simulink model "Async_3br_conv_eff"  (R2024b)
settings: Solver=ode23tb  StartTime=0.0  StopTime=10.5  MaxStep=1e-2  MinStep=1e-5  RelTol=1e-1
InitFcn:
  | sw_freq=60e3;
  | eff_rms_freq=sw_freq/10;
  | V_high=80;
  | 
  | L_ind=300e-6;
  | L_res=20e-3;
  | 
  | MOS_Ron=10e-3;
  | MOS_Vfw=1.2;
  | 
  | DIO_Vfw=0.9;
  | DIO_Ron=1e-3;
  | 
  | TRC_Res=5e-3;
  | 
  | sync_mode=1;
  | 
  | asym_bdc_p=0.01;
  | asym_bdc_i=0.8;
values from neighbouring files (symbols this model uses):
  runtime = 1.5    [compare_3d_br_ratios.m]
  timestep = runtime/size(curr_range,2)    [compare_3d_br_ratios.m]
  V_low_range = 10:5:40    [compare_3d_br_ratios.m]
undefined symbols (not defined in the file or in its folder): ratio
libraries: spsMeanLib x7, spsGroundLib x7, spsSeriesRLCBranchLib x7, slpidlib x4, spsMosfetLib x4, spsDiodeLib x2, spsStairGeneratorLib x2, spsMultimeterLib x1, spsDCVoltageSourceLib x1, spsControlledVoltageSourceLib x1, embmathops x1, spspowerguiLib x1
settings Model: SimulationMode=rapid-accelerator  Creator=adamo  LastModifiedBy=adamo
settings DebuggingCC: MaskedZcDiagnostic=none  IgnoredZcDiagnostic=none
settings HardwareCC: ProdHWDeviceType=AMD->x86-64 (Windows64)
settings RTWCC: BuildConfiguration=Faster Runs  CheckMdlBeforeBuild=Error
settings GRTTargetCC: OptimizeReductions=on
settings SimscapeCC: SimscapeCompileComponentReuse=on  SimscapeCompileArtifactsDiskCache=on

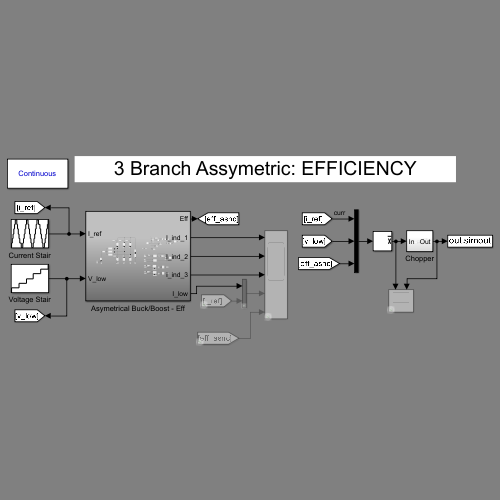
[thumbnail: Simulink's stored preview of the top-level diagram]
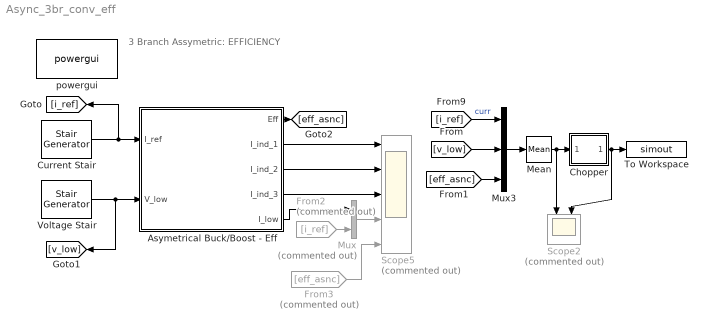
== system Async_3br_conv_eff ==
  note: 3 Branch Assymetric: EFFICIENCY
  Asymetrical Buck/Boost - Eff : Subsystem
  Chopper : Subsystem
  Current Stair : spsStairGeneratorLib/Stair Generator  t=cur_stair_time  e=current_stair  Ts=0
  From2 : From  Commented=on  GotoTag=i_ref
  From3 : From  Commented=on  GotoTag=eff_asnc
  Mean : spsMeanLib/Mean  Freq=sw_freq/10  Vinit=0  Ts=0
  Mux : Mux  Commented=on  Inputs=2
  Mux3 : Mux  Inputs=3
  Scope2 : Scope  Commented=on  NumInputPorts=2
  Scope5 : Scope  Commented=on  NumInputPorts=5
  To Workspace : ToWorkspace  VariableName=simout  SampleTime=-1
  Voltage Stair : spsStairGeneratorLib/Stair Generator  t=[0:runtime:runtime*length(V_low_range)-runtime]  e=V_low_range  Ts=0
  powergui : spspowerguiLib/powergui  Priority=1  SimulationMode=Continuous  SampleTime=50e-6  frequency=60  Iterations=50  frequencyindice=0  Pbase=100e6  ErrMax=1e-4  UnitsV=kV  UnitsW=MW  buscounter=0  FunctionMessages=off  echomessages=off  EnableUseOfTLC=off  CurrentSourceSwitches=off  DisableSnubberDevices=on  DisableRonSwitches=off  DisableVfSwitches=off  DisplayEquations=off  AutomaticDiscreteSolvers=off  SolverType=Tustin/Backward Euler (TBE)  Interpol=off  ExternalGateDelay=off  methode=on  Ts=100  x0status=blocks  SPID=on  SwTol=0  HookPort=off  NonlinearTolerance=1e-4  nMaxIteration=100  ContinueOnMaxIteration=off  RestoreLinks=warning  ResistiveCurrentMeasurement=off  Frange=[0:2:500]  Ylog=off  Xlog=on  ShowGrid=off  save=off  variable=ZData  structure=0  ZoomFFT=off  StartTime=0.0  cycles=1  DisplayStyle=1  fundamental=60  FreqAxis=off  MaxFrequency=1000  frequencyindicesteady=1  RmsSteady=1  display=off
  wires:
  Current Stair/1 -> [i_ref], Asymetrical Buck/Boost - Eff/1(I_ref)
  Asymetrical Buck/Boost - Eff/2(I_ind_1) -> Scope5/1
  Asymetrical Buck/Boost - Eff/3(I_ind_2) -> Scope5/2
  Asymetrical Buck/Boost - Eff/4(I_ind_3) -> Scope5/3
  Asymetrical Buck/Boost - Eff/1(Eff) -> [eff_asnc]
  [i_ref] -> Mux3/1  "curr"
  Mux3/1 -> Mean/1
  [eff_asnc] -> Mux3/3
  Asymetrical Buck/Boost - Eff/5(I_low) -> Mux/1
  Chopper/1(Out1) -> Scope2/2, To Workspace/1
  Mean/1 -> Scope2/1, Chopper/1(In1)
  Voltage Stair/1 -> [v_low], Asymetrical Buck/Boost - Eff/2(V_low)
  [v_low] -> Mux3/2
  Mux/1 -> Scope5/4
  From2/1 -> Mux/2
  From3/1 -> Scope5/5

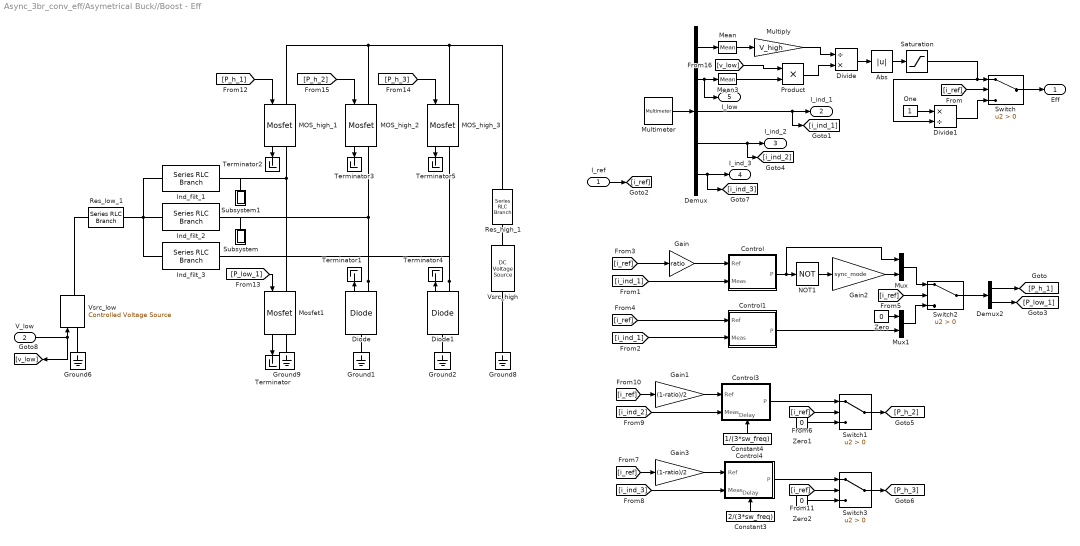
== system Async_3br_conv_eff/Asymetrical Buck//Boost - Eff ==
  I_ref : Inport
  V_low : Inport  Port=2
  Abs : Abs  SaturateOnIntegerOverflow=off
  Constant3 : Constant  Value=2/(3*sw_freq)
  Constant4 : Constant  Value=1/(3*sw_freq)
  Control : Subsystem
  Control1 : Subsystem
  Control3 : Subsystem
      settings: PortSchema="{\"entries\":[{\"content\":{\"sides\":[{\"content\":{\"connectorIds\":[\"In1\",\"In2\"]},\"type\":\"ConnectorPlacement.EquallySpacedRectSide\",\"uuid\":\"44975c06-6cb3-4b92-aa2e-c11b859d13e4\"},{\"content\":{\"connectorIds\":[\"Out1\"],\"side\":\"RIGHT\"},\"type\":\"ConnectorPlacement.EquallySpacedRectSide\",\"uuid\":\"ebdc9065-5b19-4aa7-8841-916fd82a5d31\"},{\"content\":{\"side\":\"TOP\"},\"type\":\"ConnectorPlacement.EquallySpacedRectSide\",\"uuid\":\"027925ea-888b-4bcf-b8a4-44694d0e275e\"},{\"content\":{\"connectorIds\":[\"In3\"],\"side\":\"BOTTOM\"},\"type\":\"ConnectorPlacement.EquallySpacedRectSide\",\"uuid\":\"415fb0af-dd9a-4309-9118-76332ed11379\"}]},\"type\":\"ConnectorPlacement.EquallySpacedConnector\",\"uuid\":\"3cd19595-535e-42c3-a0e6-40045bedee28\"}],\"packageUris\":[\"http://schema.mathworks.com/mf0/Connector/R2020b\"],\"version\":\"1.0\"}"
  Control4 : Subsystem
      settings: PortSchema="{\"entries\":[{\"content\":{\"sides\":[{\"content\":{\"connectorIds\":[\"In1\",\"In2\"]},\"type\":\"ConnectorPlacement.EquallySpacedRectSide\",\"uuid\":\"44975c06-6cb3-4b92-aa2e-c11b859d13e4\"},{\"content\":{\"connectorIds\":[\"Out1\"],\"side\":\"RIGHT\"},\"type\":\"ConnectorPlacement.EquallySpacedRectSide\",\"uuid\":\"ebdc9065-5b19-4aa7-8841-916fd82a5d31\"},{\"content\":{\"side\":\"TOP\"},\"type\":\"ConnectorPlacement.EquallySpacedRectSide\",\"uuid\":\"027925ea-888b-4bcf-b8a4-44694d0e275e\"},{\"content\":{\"connectorIds\":[\"In3\"],\"side\":\"BOTTOM\"},\"type\":\"ConnectorPlacement.EquallySpacedRectSide\",\"uuid\":\"9488b47a-c58c-42e9-bacd-7bb9f563b775\"}]},\"type\":\"ConnectorPlacement.EquallySpacedConnector\",\"uuid\":\"3cd19595-535e-42c3-a0e6-40045bedee28\"}],\"packageUris\":[\"http://schema.mathworks.com/mf0/Connector/R2020b\"],\"version\":\"1.0\"}"
  Demux : Demux  Outputs=5
  Demux2 : Demux  Outputs=2
  Diode : spsDiodeLib/Diode  Ron=DIO_Ron  Lon=0  Vf=DIO_Vfw  IC=0  UseSnubber=0  Rs=500  Cs=250e-9  Measurements=on
  Diode1 : spsDiodeLib/Diode  Ron=DIO_Ron  Lon=0  Vf=DIO_Vfw  IC=0  UseSnubber=0  Rs=500  Cs=250e-9  Measurements=on
  Divide : Product  Inputs=/*
  Divide1 : Product  Inputs=*/
  Gain : Gain  Gain=ratio
  Gain1 : Gain  Gain=(1-ratio)/2
  Gain2 : Gain  Gain=sync_mode  OutDataTypeStr=double
  Gain3 : Gain  Gain=(1-ratio)/2
  Ground{1..2,6,8..9} (5 alike) : spsGroundLib/Ground  LConnTagsString=a
  Ind_filt_1 : spsSeriesRLCBranchLib/Series RLC Branch  LConnTagsString=__new0  RConnTagsString=__new0  BranchType=RL  Resistance=L_res  Inductance=L_ind  SetiL0=off  InitialCurrent=0  Capacitance=1e-6  Setx0=off  InitialVoltage=0  Measurements=Branch current
  Ind_filt_2 : spsSeriesRLCBranchLib/Series RLC Branch  LConnTagsString=__new0  RConnTagsString=__new0  BranchType=RL  Resistance=L_res  Inductance=L_ind  SetiL0=off  InitialCurrent=0  Capacitance=1e-6  Setx0=off  InitialVoltage=0  Measurements=Branch current
  Ind_filt_3 : spsSeriesRLCBranchLib/Series RLC Branch  LConnTagsString=__new0  RConnTagsString=__new0  BranchType=RL  Resistance=L_res  Inductance=L_ind  SetiL0=off  InitialCurrent=0  Capacitance=1e-6  Setx0=off  InitialVoltage=0  Measurements=Branch current
  MOS_high_1 : spsMosfetLib/Mosfet  Ron=MOS_Ron  Lon=0  Rd=DIO_Ron  Vfd=MOS_Vfw  IC=0  Rs=1e5  Cs=inf  Measurements=on
  MOS_high_2 : spsMosfetLib/Mosfet  Ron=MOS_Ron  Lon=0  Rd=DIO_Ron  Vfd=MOS_Vfw  IC=0  Rs=1e5  Cs=inf  Measurements=on
  MOS_high_3 : spsMosfetLib/Mosfet  Ron=MOS_Ron  Lon=0  Rd=DIO_Ron  Vfd=MOS_Vfw  IC=0  Rs=1e5  Cs=inf  Measurements=on
  Mean : spsMeanLib/Mean  Freq=eff_rms_freq  Vinit=1  Ts=0
  Mean3 : spsMeanLib/Mean  Freq=eff_rms_freq  Vinit=1  Ts=0
  Mosfet1 : spsMosfetLib/Mosfet  Ron=MOS_Ron  Lon=0  Rd=DIO_Ron  Vfd=MOS_Vfw  IC=0  Rs=1e5  Cs=inf  Measurements=on
  Multimeter : spsMultimeterLib/Multimeter  L=5  sel=[4 5 1 2 3]  yselected={}  Gain=[1 1 1 1 1]  OutputType=Complex  PlotAtSimulationStop=off  PhasorSimulation=off
  Multiply : Gain  Gain=V_high
  Mux : Mux  Inputs=2
  Mux1 : Mux  Inputs=2
  NOT1 : Logic  Operator=NOT  IconShape=distinctive  AllPortsSameDT=off  OutDataTypeStr=boolean
  One : Constant  OutDataTypeStr=Inherit: Inherit via back propagation
  Product : Product
  Res_high_1 : spsSeriesRLCBranchLib/Series RLC Branch  LConnTagsString=__new0  RConnTagsString=__new0  BranchType=R  Resistance=TRC_Res  Inductance=1e-3  SetiL0=off  InitialCurrent=0  Capacitance=1e-6  Setx0=off  InitialVoltage=0  Measurements=Branch current
  Res_low_1 : spsSeriesRLCBranchLib/Series RLC Branch  LConnTagsString=__new0  RConnTagsString=__new0  BranchType=R  Resistance=TRC_Res  Inductance=1e-3  SetiL0=off  InitialCurrent=0  Capacitance=1e-6  Setx0=off  InitialVoltage=0  Measurements=Branch current
  Saturation : Saturate  UpperLimit=0.9999  LowerLimit=0.4
  Subsystem : Subsystem
      settings: PortSchema="{\"entries\":[{\"content\":{\"sides\":[{\"content\":{},\"type\":\"ConnectorPlacement.EquallySpacedRectSide\",\"uuid\":\"333a472d-5660-403e-9749-9e5a485a4e51\"},{\"content\":{\"side\":\"RIGHT\"},\"type\":\"ConnectorPlacement.EquallySpacedRectSide\",\"uuid\":\"46e3a3df-9b43-4056-bf49-6d97e0ff375e\"},{\"content\":{\"connectorIds\":[\"LConn1\"],\"side\":\"TOP\"},\"type\":\"ConnectorPlacement.EquallySpacedRectSide\",\"uuid\":\"a9be43b9-3284-437d-b483-2a714199e3a2\"}]},\"type\":\"ConnectorPlacement.EquallySpacedConnector\",\"uuid\":\"6030dd83-63ea-4a67-9f73-95d000b3af89\"}],\"packageUris\":[\"http://schema.mathworks.com/mf0/Connector/R2020b\"],\"version\":\"1.0\"}"
  Subsystem1 : Subsystem
      settings: PortSchema="{\"entries\":[{\"content\":{\"sides\":[{\"content\":{},\"type\":\"ConnectorPlacement.EquallySpacedRectSide\",\"uuid\":\"333a472d-5660-403e-9749-9e5a485a4e51\"},{\"content\":{\"side\":\"RIGHT\"},\"type\":\"ConnectorPlacement.EquallySpacedRectSide\",\"uuid\":\"46e3a3df-9b43-4056-bf49-6d97e0ff375e\"},{\"content\":{\"connectorIds\":[\"LConn1\"],\"side\":\"TOP\"},\"type\":\"ConnectorPlacement.EquallySpacedRectSide\",\"uuid\":\"a9be43b9-3284-437d-b483-2a714199e3a2\"}]},\"type\":\"ConnectorPlacement.EquallySpacedConnector\",\"uuid\":\"6030dd83-63ea-4a67-9f73-95d000b3af89\"}],\"packageUris\":[\"http://schema.mathworks.com/mf0/Connector/R2020b\"],\"version\":\"1.0\"}"
  Switch{,1..3} (4 alike) : Switch  Criteria=u2 > Threshold  SaturateOnIntegerOverflow=off  InputSameDT=off
  Terminator{,1..5} (6 alike) : Terminator
  Vsrc_high : spsDCVoltageSourceLib/DC Voltage Source  Amplitude=V_high  Measurements=None
  Vsrc_low : spsControlledVoltageSourceLib/Controlled Voltage Source  Initialize=on  Source_Type=DC  Amplitude=10  Phase=0  Frequency=0  Measurements=None
  Zero : Constant  Value=0  OutDataTypeStr=Inherit: Inherit via back propagation
  Zero1 : Constant  Value=0  OutDataTypeStr=Inherit: Inherit via back propagation
  Zero2 : Constant  Value=0  OutDataTypeStr=Inherit: Inherit via back propagation
  Eff : Outport
  I_ind_1 : Outport  Port=2
  I_ind_2 : Outport  Port=3
  I_ind_3 : Outport  Port=4
  I_low : Outport  Port=5
  wires:
  [P_h_1] -> MOS_high_1/1
  MOS_high_1/1 -> Terminator2/1
  Mosfet1/1 -> Terminator/1
  [P_low_1] -> Mosfet1/1
  Diode/1 -> Terminator1/1
  MOS_high_2/1 -> Terminator3/1
  Diode1/1 -> Terminator4/1
  MOS_high_3/1 -> Terminator5/1
  [P_h_3] -> MOS_high_3/1
  Multimeter/1 -> Demux/1
  One/1 -> Divide1/1
  Mean/1 -> Multiply/1
  Divide1/1 -> Switch/3
  Saturation/1 -> Divide1/2, Switch/1
  Divide/1 -> Abs/1
  Switch/1 -> Eff/1
  Abs/1 -> Saturation/1
  Control/1(P) -> Mux/1, NOT1/1
  [i_ref] -> Gain/1
  Switch2/1 -> Demux2/1
  Mux/1 -> Switch2/1
  [i_ind_1] -> Control/2(Meas)
  Demux2/2 -> [P_low_1]
  Demux2/1 -> [P_h_1]
  Gain2/1 -> Mux/2
  [i_ref] -> Switch2/2
  I_ref/1 -> [i_ref]
  [i_ref] -> Switch/2
  NOT1/1 -> Gain2/1
  [P_h_2] -> MOS_high_2/1
  Gain/1 -> Control/1(Ref)
  [i_ref] -> Control1/1(Ref)
  [i_ind_1] -> Control1/2(Meas)
  Control1/1(P) -> Mux1/2
  Mean3/1 -> Product/2
  Demux/1 -> Mean/1
  Demux/2 -> I_low/1, Mean3/1
  Demux/5 -> [i_ind_3], I_ind_3/1
  Demux/4 -> [i_ind_2], I_ind_2/1
  Demux/3 -> [i_ind_1], I_ind_1/1
  Product/1 -> Divide/2
  Multiply/1 -> Divide/1
  Mux1/1 -> Switch2/3
  Zero/1 -> Mux1/1
  Constant4/1 -> Control3/3(Delay)
  Constant3/1 -> Control4/3(Delay)
  [i_ref] -> Gain1/1
  Gain1/1 -> Control3/1(Ref)
  [i_ind_2] -> Control3/2(Meas)
  Control3/1(P) -> Switch1/1
  Switch1/1 -> [P_h_2]
  Zero1/1 -> Switch1/3
  [i_ref] -> Switch1/2
  [i_ind_3] -> Control4/2(Meas)
  [i_ref] -> Switch3/2
  Control4/1(P) -> Switch3/1
  Switch3/1 -> [P_h_3]
  Zero2/1 -> Switch3/3
  V_low/1 -> [v_low], Vsrc_low/1
  [v_low] -> Product/1
  [i_ref] -> Gain3/1
  Gain3/1 -> Control4/1(Ref)
  connections:
  Diode/RConn1 -- Ind_filt_2/LConn1 -- Subsystem/LConn1 -- MOS_high_2/RConn1
  MOS_high_1/RConn1 -- Subsystem1/LConn1 -- Ind_filt_1/LConn1 -- Mosfet1/LConn1
  Ground8/LConn1 -- Vsrc_high/LConn1
  Mosfet1/RConn1 -- Ground9/LConn1
  Vsrc_low/LConn1 -- Ground6/LConn1
  Diode/LConn1 -- Ground1/LConn1
  Diode1/RConn1 -- Ind_filt_3/LConn1 -- MOS_high_3/RConn1
  Diode1/LConn1 -- Ground2/LConn1
  Vsrc_low/RConn1 -- Res_low_1/RConn1
  Res_high_1/LConn1 -- Vsrc_high/RConn1
  Ind_filt_2/RConn1 -- Res_low_1/LConn1 -- Ind_filt_3/RConn1 -- Ind_filt_1/RConn1
  Res_high_1/RConn1 -- MOS_high_1/LConn1 -- MOS_high_2/LConn1 -- MOS_high_3/LConn1

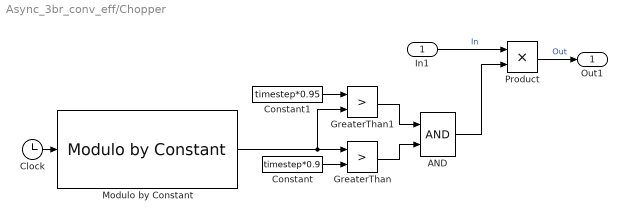
== system Async_3br_conv_eff/Chopper ==
  In1 : Inport
  AND : Logic  IconShape=distinctive  AllPortsSameDT=off  OutDataTypeStr=boolean
  Clock : Clock
  Constant : Constant  Value=timestep*0.9
  Constant1 : Constant  Value=timestep*0.95
  GreaterThan : RelationalOperator  Operator=>  OutDataTypeStr=boolean  RndMeth=Simplest  InputSameDT=off
  GreaterThan1 : RelationalOperator  Operator=>  OutDataTypeStr=boolean  RndMeth=Simplest  InputSameDT=off
  Modulo by Constant : embmathops/Modulo by Constant  Denominator=timestep  SimulateUsing=Code generation
  Product : Product
  Out1 : Outport
  wires:
  Clock/1 -> Modulo by Constant/1
  Constant/1 -> GreaterThan/2
  GreaterThan1/1 -> AND/1
  GreaterThan/1 -> AND/2
  AND/1 -> Product/2
  Modulo by Constant/1 -> GreaterThan1/2, GreaterThan/1
  Constant1/1 -> GreaterThan1/1
  In1/1 -> Product/1  "In"
  Product/1 -> Out1/1  "Out"

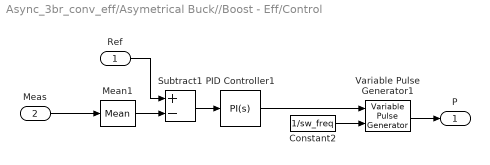
== system Async_3br_conv_eff/Asymetrical Buck//Boost - Eff/Control ==
  Ref : Inport
  Meas : Inport  Port=2
  Constant2 : Constant  Value=1/sw_freq
  Mean1 : spsMeanLib/Mean  Freq=sw_freq/10  Vinit=0  Ts=0
  PID Controller1 : slpidlib/PID Controller  Controller=PI  Form=Parallel  TimeDomain=Continuous-time  UseExternalTs=off  SampleTime=-1  IntegratorMethod=Forward Euler  FilterMethod=Forward Euler  ControllerParametersSource=internal  P=asym_bdc_p  I=asym_bdc_i  UseKiTs=on  D=0  UseExternalDerivativeSource=off  N=100  UseFilter=on  TunerSelectOption=Transfer Function Based (PID Tuner App)  InitialConditionSource=internal  InitialConditionForIntegrator=0.15  InitialConditionForFilter=0.1  DifferentiatorICPrevScaledInput=0  ExternalReset=none  TrackingMode=off  Kt=1  LimitOutput=on  SatLimitsSource=internal  UpperSaturationLimit=1  LowerSaturationLimit=0.01  LinearizeAsGain=on  AntiWindupMode=none  Kb=1  LimitIntegrator=off  UpperIntegratorSaturationLimit=inf  LowerIntegratorSaturationLimit=-inf  POutMin=[]  POutMax=[]  IOutMin=[]  IOutMax=[]  DOutMin=[]  DOutMax=[]  NOutMin=[]  NOutMax=[]  SumOutMin=[]  SumOutMax=[]  SaturationOutMin=[]  SaturationOutMax=[]  PParamMin=[]  PParamMax=[]  IParamMin=[]  IParamMax=[]  DParamMin=[]  DParamMax=[]  NParamMin=[]  NParamMax=[]  KbParamMin=[]  KbParamMax=[]  KtParamMin=[]  KtParamMax=[]  KbOutMin=[]  KbOutMax=[]  KtOutMin=[]  KtOutMax=[]  IntegratorOutMin=[]  IntegratorOutMax=[]  FilterOutMin=[]  FilterOutMax=[]  SumI1OutMin=[]  SumI1OutMax=[]  SumI2OutMin=[]  SumI2OutMax=[]  SumI3OutMin=[]  SumI3OutMax=[]  SumI4OutMin=[]  SumI4OutMax=[]  SumDOutMin=[]  SumDOutMax=[]  DifferentiatorOutMin=[]  DifferentiatorOutMax=[]  FilterDiffOutCoefMin=[]  FilterDiffOutCoefMax=[]  ReciprocalOutMin=[]  ReciprocalOutMax=[]  SumDenOutMin=[]  SumDenOutMax=[]  SumNumOutMin=[]  SumNumOutMax=[]  DivideOutMin=[]  DivideOutMax=[]  UdiffTsProdOutMin=[]  UdiffTsProdOutMax=[]  NTsProdOutMin=[]  NTsProdOutMax=[]  UintegralTsProdOutMin=[]  UintegralTsProdOutMax=[]  UngainTsProdOutMin=[]  UngainTsProdOutMax=[]  ClampingZeroOutDataTypeStr=Inherit: Inherit via back propagation  ClampingZeroOutMin=[]  ClampingZeroOutMax=[]  FilterDenConstantOutDataTypeStr=Inherit: Inherit via back propagation  FilterDenConstantOutMin=[]  FilterDenConstantOutMax=[]  PCopyOutDataTypeStr=Inherit: Inherit via back propagation  PCopyOutMin=[]  PCopyOutMax=[]  NCopyOutDataTypeStr=Inherit: Inherit via back propagation  NCopyOutMin=[]  NCopyOutMax=[]  IntegratorContinuousStateAttributes=''  IntegratorStateMustResolveToSignalObject=off  IntegratorRTWStateStorageClass=Auto  FilterContinuousStateAttributes=''  FilterStateMustResolveToSignalObject=off  FilterRTWStateStorageClass=Auto  ParallelPVariant=InternalParameters  IdealPVariant=Disabled  IVariant=InternalParameters  DVariant=Disabled  IntegratorVariant=Continuous  SatVariant=Enabled  AWVariant=Passthrough  PCopyVariant=Disabled  TRVariant=Disabled  FdbkBlocksVariant=Forward  IdealPFdbkVariant=Disabled  SatFdbkVariant=Disabled  DerivativeFilterVariant=Disabled  NVariant=Disabled  NCopyVariant=Disabled_SignalSpec  FilterICVariant=Disabled  IntegratorICVariant=InternalICs  ExternalResetVariant=Disabled  TRSumVariant=Passthrough  SumFdbkVariant=Disabled  SumVariant=Sum_PI  TsampFilterVariant=InternalTs  TsampNgainVariant=Passthrough  TsampIntegralVariant=Disabled_SignalSpec  ExternalSaturationOutDataTypeStr=Inherit: Same as second input  DerivativeSourceVariant=Disabled  PreIntVariant=InternalPreInt
  Subtract1 : Sum  Inputs=+-
  Variable Pulse Generator1 : VariablePulseGenerator  AllowZeroPulseWidth=on  SampleTime=0.1
  P : Outport
  wires:
  Meas/1 -> Mean1/1
  PID Controller1/1 -> Variable Pulse Generator1/1
  Constant2/1 -> Variable Pulse Generator1/2
  Mean1/1 -> Subtract1/2
  Subtract1/1 -> PID Controller1/1
  Variable Pulse Generator1/1 -> P/1
  Ref/1 -> Subtract1/1

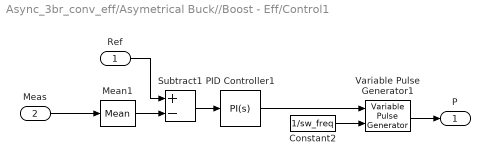
== system Async_3br_conv_eff/Asymetrical Buck//Boost - Eff/Control1 ==
  Ref : Inport
  Meas : Inport  Port=2
  Constant2 : Constant  Value=1/sw_freq
  Mean1 : spsMeanLib/Mean  Freq=sw_freq/10  Vinit=0  Ts=0
  PID Controller1 : slpidlib/PID Controller  Controller=PI  Form=Parallel  TimeDomain=Continuous-time  UseExternalTs=off  SampleTime=-1  IntegratorMethod=Forward Euler  FilterMethod=Forward Euler  ControllerParametersSource=internal  P=asym_bdc_p  I=asym_bdc_i  UseKiTs=on  D=0  UseExternalDerivativeSource=off  N=100  UseFilter=on  TunerSelectOption=Transfer Function Based (PID Tuner App)  InitialConditionSource=internal  InitialConditionForIntegrator=0  InitialConditionForFilter=0  DifferentiatorICPrevScaledInput=0  ExternalReset=none  TrackingMode=off  Kt=1  LimitOutput=on  SatLimitsSource=internal  UpperSaturationLimit=1  LowerSaturationLimit=0  LinearizeAsGain=on  AntiWindupMode=none  Kb=1  LimitIntegrator=off  UpperIntegratorSaturationLimit=inf  LowerIntegratorSaturationLimit=-inf  POutMin=[]  POutMax=[]  IOutMin=[]  IOutMax=[]  DOutMin=[]  DOutMax=[]  NOutMin=[]  NOutMax=[]  SumOutMin=[]  SumOutMax=[]  SaturationOutMin=[]  SaturationOutMax=[]  PParamMin=[]  PParamMax=[]  IParamMin=[]  IParamMax=[]  DParamMin=[]  DParamMax=[]  NParamMin=[]  NParamMax=[]  KbParamMin=[]  KbParamMax=[]  KtParamMin=[]  KtParamMax=[]  KbOutMin=[]  KbOutMax=[]  KtOutMin=[]  KtOutMax=[]  IntegratorOutMin=[]  IntegratorOutMax=[]  FilterOutMin=[]  FilterOutMax=[]  SumI1OutMin=[]  SumI1OutMax=[]  SumI2OutMin=[]  SumI2OutMax=[]  SumI3OutMin=[]  SumI3OutMax=[]  SumI4OutMin=[]  SumI4OutMax=[]  SumDOutMin=[]  SumDOutMax=[]  DifferentiatorOutMin=[]  DifferentiatorOutMax=[]  FilterDiffOutCoefMin=[]  FilterDiffOutCoefMax=[]  ReciprocalOutMin=[]  ReciprocalOutMax=[]  SumDenOutMin=[]  SumDenOutMax=[]  SumNumOutMin=[]  SumNumOutMax=[]  DivideOutMin=[]  DivideOutMax=[]  UdiffTsProdOutMin=[]  UdiffTsProdOutMax=[]  NTsProdOutMin=[]  NTsProdOutMax=[]  UintegralTsProdOutMin=[]  UintegralTsProdOutMax=[]  UngainTsProdOutMin=[]  UngainTsProdOutMax=[]  ClampingZeroOutDataTypeStr=Inherit: Inherit via back propagation  ClampingZeroOutMin=[]  ClampingZeroOutMax=[]  FilterDenConstantOutDataTypeStr=Inherit: Inherit via back propagation  FilterDenConstantOutMin=[]  FilterDenConstantOutMax=[]  PCopyOutDataTypeStr=Inherit: Inherit via back propagation  PCopyOutMin=[]  PCopyOutMax=[]  NCopyOutDataTypeStr=Inherit: Inherit via back propagation  NCopyOutMin=[]  NCopyOutMax=[]  IntegratorContinuousStateAttributes=''  IntegratorStateMustResolveToSignalObject=off  IntegratorRTWStateStorageClass=Auto  FilterContinuousStateAttributes=''  FilterStateMustResolveToSignalObject=off  FilterRTWStateStorageClass=Auto  ParallelPVariant=InternalParameters  IdealPVariant=Disabled  IVariant=InternalParameters  DVariant=Disabled  IntegratorVariant=Continuous  SatVariant=Enabled  AWVariant=Passthrough  PCopyVariant=Disabled  TRVariant=Disabled  FdbkBlocksVariant=Forward  IdealPFdbkVariant=Disabled  SatFdbkVariant=Disabled  DerivativeFilterVariant=Disabled  NVariant=Disabled  NCopyVariant=Disabled_SignalSpec  FilterICVariant=Disabled  IntegratorICVariant=InternalICs  ExternalResetVariant=Disabled  TRSumVariant=Passthrough  SumFdbkVariant=Disabled  SumVariant=Sum_PI  TsampFilterVariant=InternalTs  TsampNgainVariant=Passthrough  TsampIntegralVariant=Disabled_SignalSpec  ExternalSaturationOutDataTypeStr=Inherit: Same as second input  DerivativeSourceVariant=Disabled  PreIntVariant=InternalPreInt
  Subtract1 : Sum  Inputs=+-
  Variable Pulse Generator1 : VariablePulseGenerator  AllowZeroPulseWidth=on  SampleTime=0.1
  P : Outport
  wires:
  Meas/1 -> Mean1/1
  PID Controller1/1 -> Variable Pulse Generator1/1
  Constant2/1 -> Variable Pulse Generator1/2
  Mean1/1 -> Subtract1/2
  Subtract1/1 -> PID Controller1/1
  Variable Pulse Generator1/1 -> P/1
  Ref/1 -> Subtract1/1

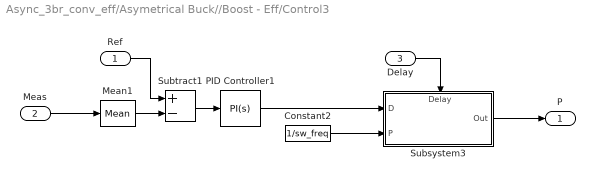
== system Async_3br_conv_eff/Asymetrical Buck//Boost - Eff/Control3 ==
  Ref : Inport
  Meas : Inport  Port=2
  Delay : Inport  Port=3
  Constant2 : Constant  Value=1/sw_freq
  Mean1 : spsMeanLib/Mean  Freq=sw_freq/10  Vinit=0  Ts=0
  PID Controller1 : slpidlib/PID Controller  Controller=PI  Form=Parallel  TimeDomain=Continuous-time  UseExternalTs=off  SampleTime=-1  IntegratorMethod=Forward Euler  FilterMethod=Forward Euler  ControllerParametersSource=internal  P=asym_bdc_p  I=asym_bdc_i  UseKiTs=on  D=0  UseExternalDerivativeSource=off  N=100  UseFilter=on  TunerSelectOption=Transfer Function Based (PID Tuner App)  InitialConditionSource=internal  InitialConditionForIntegrator=0.15  InitialConditionForFilter=0.1  DifferentiatorICPrevScaledInput=0  ExternalReset=none  TrackingMode=off  Kt=1  LimitOutput=on  SatLimitsSource=internal  UpperSaturationLimit=1  LowerSaturationLimit=0.01  LinearizeAsGain=on  AntiWindupMode=none  Kb=1  LimitIntegrator=off  UpperIntegratorSaturationLimit=inf  LowerIntegratorSaturationLimit=-inf  POutMin=[]  POutMax=[]  IOutMin=[]  IOutMax=[]  DOutMin=[]  DOutMax=[]  NOutMin=[]  NOutMax=[]  SumOutMin=[]  SumOutMax=[]  SaturationOutMin=[]  SaturationOutMax=[]  PParamMin=[]  PParamMax=[]  IParamMin=[]  IParamMax=[]  DParamMin=[]  DParamMax=[]  NParamMin=[]  NParamMax=[]  KbParamMin=[]  KbParamMax=[]  KtParamMin=[]  KtParamMax=[]  KbOutMin=[]  KbOutMax=[]  KtOutMin=[]  KtOutMax=[]  IntegratorOutMin=[]  IntegratorOutMax=[]  FilterOutMin=[]  FilterOutMax=[]  SumI1OutMin=[]  SumI1OutMax=[]  SumI2OutMin=[]  SumI2OutMax=[]  SumI3OutMin=[]  SumI3OutMax=[]  SumI4OutMin=[]  SumI4OutMax=[]  SumDOutMin=[]  SumDOutMax=[]  DifferentiatorOutMin=[]  DifferentiatorOutMax=[]  FilterDiffOutCoefMin=[]  FilterDiffOutCoefMax=[]  ReciprocalOutMin=[]  ReciprocalOutMax=[]  SumDenOutMin=[]  SumDenOutMax=[]  SumNumOutMin=[]  SumNumOutMax=[]  DivideOutMin=[]  DivideOutMax=[]  UdiffTsProdOutMin=[]  UdiffTsProdOutMax=[]  NTsProdOutMin=[]  NTsProdOutMax=[]  UintegralTsProdOutMin=[]  UintegralTsProdOutMax=[]  UngainTsProdOutMin=[]  UngainTsProdOutMax=[]  ClampingZeroOutDataTypeStr=Inherit: Inherit via back propagation  ClampingZeroOutMin=[]  ClampingZeroOutMax=[]  FilterDenConstantOutDataTypeStr=Inherit: Inherit via back propagation  FilterDenConstantOutMin=[]  FilterDenConstantOutMax=[]  PCopyOutDataTypeStr=Inherit: Inherit via back propagation  PCopyOutMin=[]  PCopyOutMax=[]  NCopyOutDataTypeStr=Inherit: Inherit via back propagation  NCopyOutMin=[]  NCopyOutMax=[]  IntegratorContinuousStateAttributes=''  IntegratorStateMustResolveToSignalObject=off  IntegratorRTWStateStorageClass=Auto  FilterContinuousStateAttributes=''  FilterStateMustResolveToSignalObject=off  FilterRTWStateStorageClass=Auto  ParallelPVariant=InternalParameters  IdealPVariant=Disabled  IVariant=InternalParameters  DVariant=Disabled  IntegratorVariant=Continuous  SatVariant=Enabled  AWVariant=Passthrough  PCopyVariant=Disabled  TRVariant=Disabled  FdbkBlocksVariant=Forward  IdealPFdbkVariant=Disabled  SatFdbkVariant=Disabled  DerivativeFilterVariant=Disabled  NVariant=Disabled  NCopyVariant=Disabled_SignalSpec  FilterICVariant=Disabled  IntegratorICVariant=InternalICs  ExternalResetVariant=Disabled  TRSumVariant=Passthrough  SumFdbkVariant=Disabled  SumVariant=Sum_PI  TsampFilterVariant=InternalTs  TsampNgainVariant=Passthrough  TsampIntegralVariant=Disabled_SignalSpec  ExternalSaturationOutDataTypeStr=Inherit: Same as second input  DerivativeSourceVariant=Disabled  PreIntVariant=InternalPreInt
  Subsystem3 : Subsystem
      settings: PortSchema="{\"entries\":[{\"content\":{\"sides\":[{\"content\":{\"connectorIds\":[\"In1\",\"In2\"]},\"type\":\"ConnectorPlacement.EquallySpacedRectSide\",\"uuid\":\"51b045c8-d819-4b7c-a29d-1a54f5fd995d\"},{\"content\":{\"connectorIds\":[\"Out1\"],\"side\":\"RIGHT\"},\"type\":\"ConnectorPlacement.EquallySpacedRectSide\",\"uuid\":\"9f0647dc-9c35-4883-9e64-6da00897cce8\"},{\"content\":{\"connectorIds\":[\"In3\"],\"side\":\"TOP\"},\"type\":\"ConnectorPlacement.EquallySpacedRectSide\",\"uuid\":\"a4aa7abf-9a58-441d-bef7-3a2aafbde944\"}]},\"type\":\"ConnectorPlacement.EquallySpacedConnector\",\"uuid\":\"237ebc79-3794-4318-8db8-2d16dc313947\"}],\"packageUris\":[\"http://schema.mathworks.com/mf0/Connector/R2020b\"],\"version\":\"1.0\"}"
  Subtract1 : Sum  Inputs=+-
  P : Outport
  wires:
  Meas/1 -> Mean1/1
  Mean1/1 -> Subtract1/2
  Subtract1/1 -> PID Controller1/1
  Ref/1 -> Subtract1/1
  Delay/1 -> Subsystem3/3(Delay)
  PID Controller1/1 -> Subsystem3/1(D)
  Constant2/1 -> Subsystem3/2(P)
  Subsystem3/1(Out) -> P/1

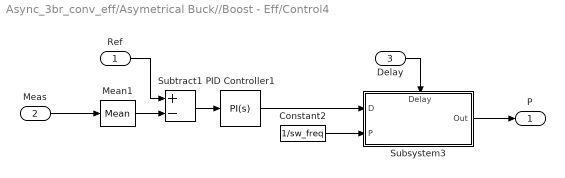
== system Async_3br_conv_eff/Asymetrical Buck//Boost - Eff/Control4 ==
  Ref : Inport
  Meas : Inport  Port=2
  Delay : Inport  Port=3
  Constant2 : Constant  Value=1/sw_freq
  Mean1 : spsMeanLib/Mean  Freq=sw_freq/10  Vinit=0  Ts=0
  PID Controller1 : slpidlib/PID Controller  Controller=PI  Form=Parallel  TimeDomain=Continuous-time  UseExternalTs=off  SampleTime=-1  IntegratorMethod=Forward Euler  FilterMethod=Forward Euler  ControllerParametersSource=internal  P=asym_bdc_p  I=asym_bdc_i  UseKiTs=on  D=0  UseExternalDerivativeSource=off  N=100  UseFilter=on  TunerSelectOption=Transfer Function Based (PID Tuner App)  InitialConditionSource=internal  InitialConditionForIntegrator=0.15  InitialConditionForFilter=0.1  DifferentiatorICPrevScaledInput=0  ExternalReset=none  TrackingMode=off  Kt=1  LimitOutput=on  SatLimitsSource=internal  UpperSaturationLimit=1  LowerSaturationLimit=0.01  LinearizeAsGain=on  AntiWindupMode=none  Kb=1  LimitIntegrator=off  UpperIntegratorSaturationLimit=inf  LowerIntegratorSaturationLimit=-inf  POutMin=[]  POutMax=[]  IOutMin=[]  IOutMax=[]  DOutMin=[]  DOutMax=[]  NOutMin=[]  NOutMax=[]  SumOutMin=[]  SumOutMax=[]  SaturationOutMin=[]  SaturationOutMax=[]  PParamMin=[]  PParamMax=[]  IParamMin=[]  IParamMax=[]  DParamMin=[]  DParamMax=[]  NParamMin=[]  NParamMax=[]  KbParamMin=[]  KbParamMax=[]  KtParamMin=[]  KtParamMax=[]  KbOutMin=[]  KbOutMax=[]  KtOutMin=[]  KtOutMax=[]  IntegratorOutMin=[]  IntegratorOutMax=[]  FilterOutMin=[]  FilterOutMax=[]  SumI1OutMin=[]  SumI1OutMax=[]  SumI2OutMin=[]  SumI2OutMax=[]  SumI3OutMin=[]  SumI3OutMax=[]  SumI4OutMin=[]  SumI4OutMax=[]  SumDOutMin=[]  SumDOutMax=[]  DifferentiatorOutMin=[]  DifferentiatorOutMax=[]  FilterDiffOutCoefMin=[]  FilterDiffOutCoefMax=[]  ReciprocalOutMin=[]  ReciprocalOutMax=[]  SumDenOutMin=[]  SumDenOutMax=[]  SumNumOutMin=[]  SumNumOutMax=[]  DivideOutMin=[]  DivideOutMax=[]  UdiffTsProdOutMin=[]  UdiffTsProdOutMax=[]  NTsProdOutMin=[]  NTsProdOutMax=[]  UintegralTsProdOutMin=[]  UintegralTsProdOutMax=[]  UngainTsProdOutMin=[]  UngainTsProdOutMax=[]  ClampingZeroOutDataTypeStr=Inherit: Inherit via back propagation  ClampingZeroOutMin=[]  ClampingZeroOutMax=[]  FilterDenConstantOutDataTypeStr=Inherit: Inherit via back propagation  FilterDenConstantOutMin=[]  FilterDenConstantOutMax=[]  PCopyOutDataTypeStr=Inherit: Inherit via back propagation  PCopyOutMin=[]  PCopyOutMax=[]  NCopyOutDataTypeStr=Inherit: Inherit via back propagation  NCopyOutMin=[]  NCopyOutMax=[]  IntegratorContinuousStateAttributes=''  IntegratorStateMustResolveToSignalObject=off  IntegratorRTWStateStorageClass=Auto  FilterContinuousStateAttributes=''  FilterStateMustResolveToSignalObject=off  FilterRTWStateStorageClass=Auto  ParallelPVariant=InternalParameters  IdealPVariant=Disabled  IVariant=InternalParameters  DVariant=Disabled  IntegratorVariant=Continuous  SatVariant=Enabled  AWVariant=Passthrough  PCopyVariant=Disabled  TRVariant=Disabled  FdbkBlocksVariant=Forward  IdealPFdbkVariant=Disabled  SatFdbkVariant=Disabled  DerivativeFilterVariant=Disabled  NVariant=Disabled  NCopyVariant=Disabled_SignalSpec  FilterICVariant=Disabled  IntegratorICVariant=InternalICs  ExternalResetVariant=Disabled  TRSumVariant=Passthrough  SumFdbkVariant=Disabled  SumVariant=Sum_PI  TsampFilterVariant=InternalTs  TsampNgainVariant=Passthrough  TsampIntegralVariant=Disabled_SignalSpec  ExternalSaturationOutDataTypeStr=Inherit: Same as second input  DerivativeSourceVariant=Disabled  PreIntVariant=InternalPreInt
  Subsystem3 : Subsystem
      settings: PortSchema="{\"entries\":[{\"content\":{\"sides\":[{\"content\":{\"connectorIds\":[\"In1\",\"In2\"]},\"type\":\"ConnectorPlacement.EquallySpacedRectSide\",\"uuid\":\"51b045c8-d819-4b7c-a29d-1a54f5fd995d\"},{\"content\":{\"connectorIds\":[\"Out1\"],\"side\":\"RIGHT\"},\"type\":\"ConnectorPlacement.EquallySpacedRectSide\",\"uuid\":\"9f0647dc-9c35-4883-9e64-6da00897cce8\"},{\"content\":{\"connectorIds\":[\"In3\"],\"side\":\"TOP\"},\"type\":\"ConnectorPlacement.EquallySpacedRectSide\",\"uuid\":\"a4aa7abf-9a58-441d-bef7-3a2aafbde944\"}]},\"type\":\"ConnectorPlacement.EquallySpacedConnector\",\"uuid\":\"237ebc79-3794-4318-8db8-2d16dc313947\"}],\"packageUris\":[\"http://schema.mathworks.com/mf0/Connector/R2020b\"],\"version\":\"1.0\"}"
  Subtract1 : Sum  Inputs=+-
  P : Outport
  wires:
  Meas/1 -> Mean1/1
  Mean1/1 -> Subtract1/2
  Subtract1/1 -> PID Controller1/1
  Subsystem3/1(Out) -> P/1
  Ref/1 -> Subtract1/1
  Constant2/1 -> Subsystem3/2(P)
  Delay/1 -> Subsystem3/3(Delay)
  PID Controller1/1 -> Subsystem3/1(D)

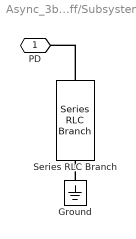
== system Async_3br_conv_eff/Asymetrical Buck//Boost - Eff/Subsystem ==
  Ground : spsGroundLib/Ground  LConnTagsString=a
  Series RLC Branch : spsSeriesRLCBranchLib/Series RLC Branch  LConnTagsString=__new0  RConnTagsString=__new0  BranchType=R  Resistance=1e6  Inductance=1e-3  SetiL0=off  InitialCurrent=0  Capacitance=1e-6  Setx0=off  InitialVoltage=0  Measurements=None
  PD : PMIOPort  Side=Left
  connections:
  Ground/LConn1 -- Series RLC Branch/RConn1
  Series RLC Branch/LConn1 -- PD/RConn1

== system Async_3br_conv_eff/Asymetrical Buck//Boost - Eff/Subsystem1 ==
  Ground : spsGroundLib/Ground  LConnTagsString=a
  Series RLC Branch : spsSeriesRLCBranchLib/Series RLC Branch  LConnTagsString=__new0  RConnTagsString=__new0  BranchType=R  Resistance=1e6  Inductance=1e-3  SetiL0=off  InitialCurrent=0  Capacitance=1e-6  Setx0=off  InitialVoltage=0  Measurements=None
  PD : PMIOPort  Side=Left
  connections:
  Ground/LConn1 -- Series RLC Branch/RConn1
  Series RLC Branch/LConn1 -- PD/RConn1

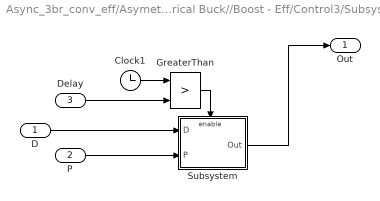
== system Async_3br_conv_eff/Asymetrical Buck//Boost - Eff/Control3/Subsystem3 ==
  D : Inport
  P : Inport  Port=2
  Delay : Inport  Port=3
  Clock1 : Clock
  GreaterThan : RelationalOperator  Operator=>  OutDataTypeStr=boolean  RndMeth=Simplest  InputSameDT=off
  Subsystem : Subsystem
  Out : Outport
  wires:
  Clock1/1 -> GreaterThan/1
  P/1 -> Subsystem/2(P)
  GreaterThan/1 -> Subsystem/Enable
  D/1 -> Subsystem/1(D)
  Delay/1 -> GreaterThan/2
  Subsystem/1(Out) -> Out/1

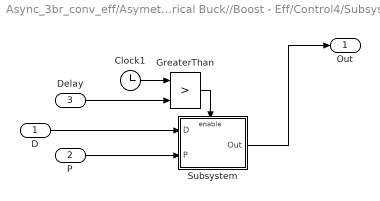
== system Async_3br_conv_eff/Asymetrical Buck//Boost - Eff/Control4/Subsystem3 ==
  D : Inport
  P : Inport  Port=2
  Delay : Inport  Port=3
  Clock1 : Clock
  GreaterThan : RelationalOperator  Operator=>  OutDataTypeStr=boolean  RndMeth=Simplest  InputSameDT=off
  Subsystem : Subsystem
  Out : Outport
  wires:
  Clock1/1 -> GreaterThan/1
  P/1 -> Subsystem/2(P)
  GreaterThan/1 -> Subsystem/Enable
  D/1 -> Subsystem/1(D)
  Delay/1 -> GreaterThan/2
  Subsystem/1(Out) -> Out/1

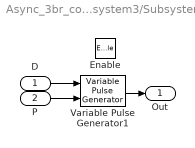
== system Async_3br_conv_eff/Asymetrical Buck//Boost - Eff/Control3/Subsystem3/Subsystem ==
  D : Inport
  P : Inport  Port=2
  Enable : EnablePort
  Variable Pulse Generator1 : VariablePulseGenerator  AllowZeroPulseWidth=on  SampleTime=0.1
  Out : Outport
  wires:
  D/1 -> Variable Pulse Generator1/1
  Variable Pulse Generator1/1 -> Out/1
  P/1 -> Variable Pulse Generator1/2

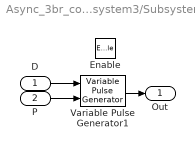
== system Async_3br_conv_eff/Asymetrical Buck//Boost - Eff/Control4/Subsystem3/Subsystem ==
  D : Inport
  P : Inport  Port=2
  Enable : EnablePort
  Variable Pulse Generator1 : VariablePulseGenerator  AllowZeroPulseWidth=on  SampleTime=0.1
  Out : Outport
  wires:
  D/1 -> Variable Pulse Generator1/1
  Variable Pulse Generator1/1 -> Out/1
  P/1 -> Variable Pulse Generator1/2
